simulink subsystem "MPU_SubSystem"  (R2021a)
settings: Solver=VariableStepAuto  StartTime=0.0  StopTime=10.0  RelTol=1e-3
undefined symbols (not defined in the file): g, ms22g, sens, Ts, wheel
settings Model: Creator=utente-A  LastModifiedBy=utente-A

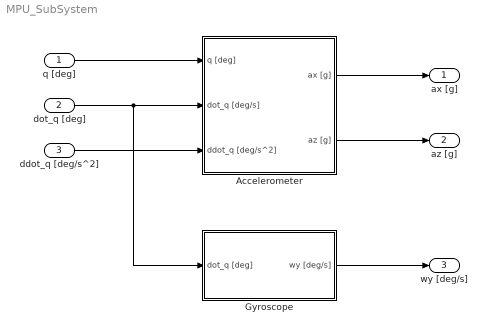
== system MPU_SubSystem ==
  q [deg] : Inport
  dot_q [deg] : Inport  Port=2
  ddot_q [deg/s^2] : Inport  Port=3
  Accelerometer : Subsystem
  Gyroscope : Subsystem
  ax [g] : Outport
  az [g] : Outport  Port=2
  wy [deg/s] : Outport  Port=3
  wires:
  Gyroscope/1(wy [deg/s]) -> wy [deg/s]/1
  Accelerometer/2(az [g]) -> az [g]/1
  Accelerometer/1(ax [g]) -> ax [g]/1
  ddot_q [deg/s^2]/1 -> Accelerometer/3(ddot_q [deg/s^2])
  q [deg]/1 -> Accelerometer/1(q [deg])
  dot_q [deg]/1 -> Accelerometer/2(dot_q [deg/s]), Gyroscope/1(dot_q [deg])

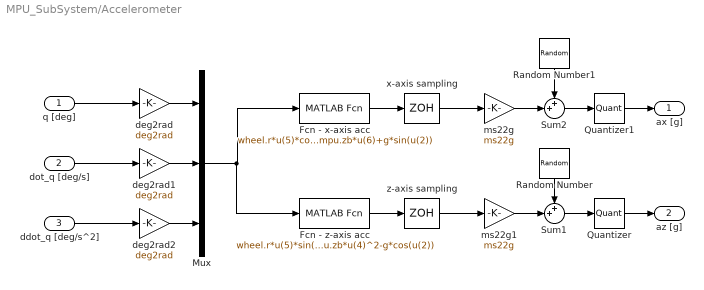
== system MPU_SubSystem/Accelerometer ==
  q [deg] : Inport
  dot_q [deg/s] : Inport  Port=2
  ddot_q [deg/s^2] : Inport  Port=3
  Fcn - x-axis acc : MATLABFcn  MATLABFcn=wheel.r*u(5)*cos(u(2))+sens.mpu.zb*u(6)+g*sin(u(2))
  Fcn - z-axis acc : MATLABFcn  MATLABFcn=wheel.r*u(5)*sin(u(2))-sens.mpu.zb*u(4)^2-g*cos(u(2))
  Mux : Mux  Inputs=3
  Quantizer : Quantizer  QuantizationInterval=sens.mpu.acc.LSB2g
  Quantizer1 : Quantizer  QuantizationInterval=sens.mpu.acc.LSB2g
  Random Number : RandomNumber  Variance=sens.mpu.acc.noisevar  SampleTime=Ts
  Random Number1 : RandomNumber  Variance=sens.mpu.acc.noisevar  SampleTime=Ts
  Sum1 : Sum  Inputs=++|
  Sum2 : Sum  Inputs=++|
  deg2rad : Gain  Gain=deg2rad
  deg2rad1 : Gain  Gain=deg2rad
  deg2rad2 : Gain  Gain=deg2rad
  ms22g : Gain  Gain=ms22g
  ms22g1 : Gain  Gain=ms22g
  x-axis sampling : ZeroOrderHold  SampleTime=Ts
  z-axis sampling : ZeroOrderHold  SampleTime=Ts
  ax [g] : Outport
  az [g] : Outport  Port=2
  wires:
  dot_q [deg/s]/1 -> deg2rad1/1
  deg2rad/1 -> Mux/1
  Mux/1 -> Fcn - x-axis acc/1, Fcn - z-axis acc/1
  Quantizer/1 -> az [g]/1
  Random Number/1 -> Sum1/1
  Random Number1/1 -> Sum2/1
  z-axis sampling/1 -> ms22g1/1
  Sum1/1 -> Quantizer/1
  q [deg]/1 -> deg2rad/1
  Quantizer1/1 -> ax [g]/1
  Sum2/1 -> Quantizer1/1
  ddot_q [deg/s^2]/1 -> deg2rad2/1
  deg2rad1/1 -> Mux/2
  deg2rad2/1 -> Mux/3
  ms22g/1 -> Sum2/2
  Fcn - x-axis acc/1 -> x-axis sampling/1
  Fcn - z-axis acc/1 -> z-axis sampling/1
  x-axis sampling/1 -> ms22g/1
  ms22g1/1 -> Sum1/2

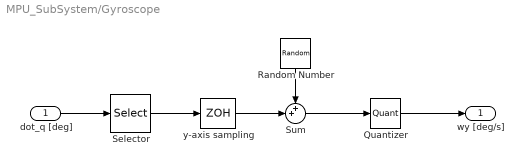
== system MPU_SubSystem/Gyroscope ==
  dot_q [deg] : Inport
  Quantizer : Quantizer  QuantizationInterval=sens.mpu.gyro.LSB2degs
  Random Number : RandomNumber  Variance=sens.mpu.gyro.noisevar  SampleTime=Ts
  Selector : Selector  InputPortWidth=2  IndexOptions=Index vector (dialog)  Indices=[2]  OutputSizes=1
  Sum : Sum  Inputs=++|
  y-axis sampling : ZeroOrderHold  SampleTime=Ts
  wy [deg/s] : Outport
  wires:
  Quantizer/1 -> wy [deg/s]/1
  Random Number/1 -> Sum/1
  y-axis sampling/1 -> Sum/2
  dot_q [deg]/1 -> Selector/1
  Selector/1 -> y-axis sampling/1
  Sum/1 -> Quantizer/1
